simulink model "PWM_Sawtooth"  (R2015b)
settings: Solver=VariableStepAuto  StartTime=0.0  StopTime=1  RelTol=1e-3
libraries: powerlib_meascontrol x2
settings Model: Creator=akhta  LastModifiedBy=akhta

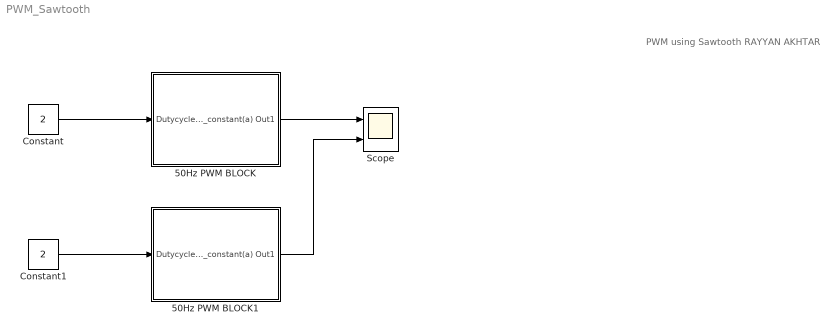
== system PWM_Sawtooth ==
  note: PWM using Sawtooth
      |
      | RAYYAN AKHTAR
  50Hz PWM BLOCK : Subsystem
  50Hz PWM BLOCK1 : Subsystem
  Constant : Constant  Value=2
  Constant1 : Constant  Value=2
  Scope : Scope  NumInputPorts=2
  wires:
  Constant/1 -> 50Hz PWM BLOCK/1(Dutycycle_constant(a))
  50Hz PWM BLOCK/1(Out1) -> Scope/1
  Constant1/1 -> 50Hz PWM BLOCK1/1(Dutycycle_constant(a))
  50Hz PWM BLOCK1/1(Out1) -> Scope/2

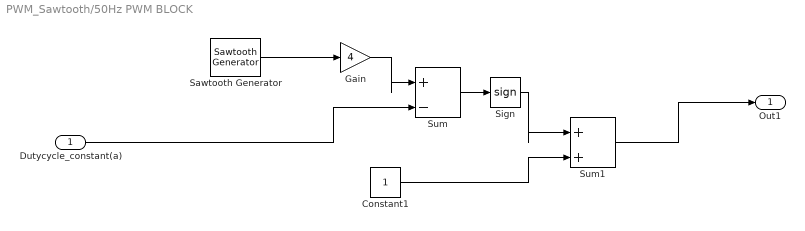
== system PWM_Sawtooth/50Hz PWM BLOCK ==
  Dutycycle_constant(a) : Inport
  Constant1 : Constant
  Gain : Gain  Gain=4
  Sawtooth Generator : powerlib_meascontrol/Pulse & Signal Generators/Sawtooth Generator  Freq=25e3  Phase=0  Ts=0
  Sign : Signum
  Sum : Sum  Inputs=|+-
  Sum1 : Sum  Inputs=|++
  Out1 : Outport
  wires:
  Sum1/1 -> Out1/1
  Gain/1 -> Sum/1
  Sign/1 -> Sum1/1
  Constant1/1 -> Sum1/2
  Sum/1 -> Sign/1
  Sawtooth Generator/1 -> Gain/1
  Dutycycle_constant(a)/1 -> Sum/2

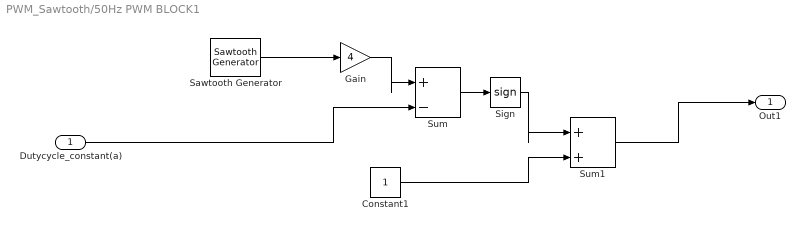
== system PWM_Sawtooth/50Hz PWM BLOCK1 ==
  Dutycycle_constant(a) : Inport
  Constant1 : Constant
  Gain : Gain  Gain=4
  Sawtooth Generator : powerlib_meascontrol/Pulse & Signal Generators/Sawtooth Generator  Freq=25e3  Phase=-90  Ts=0
  Sign : Signum
  Sum : Sum  Inputs=|+-
  Sum1 : Sum  Inputs=|++
  Out1 : Outport
  wires:
  Sum1/1 -> Out1/1
  Gain/1 -> Sum/1
  Sign/1 -> Sum1/1
  Constant1/1 -> Sum1/2
  Sum/1 -> Sign/1
  Sawtooth Generator/1 -> Gain/1
  Dutycycle_constant(a)/1 -> Sum/2
